simulink model "Design_5new_4weeks"  (R2026a)
settings: Solver=FixedStepAuto  StopTime=200000  FixedStep=300
undefined symbols (not defined in the file): m, n
libraries: mqttlib x7
(part 2 of 2)

== matlab function Design_5new_4weeks/MATLAB Function 3 ==
  data: t input; dt output



function dt = fcn_printer2(t)
%#codegen

SEC_PER_DAY = 24*3600;
rel_sec = 8*3600;    % Same as Printer 1 → 08:00 AM
epsT = 1e-9;

day  = floor(t/SEC_PER_DAY);
tod  = mod(t, SEC_PER_DAY);

next_day = day;

while true
    ndow  = mod(next_day,7);      % day of week
    nweek = floor(next_day/7);    % week index

    % Skip weekends
    if ndow == 5 || ndow == 6
        next_day = next_day + 1;
        continue;
    end

    % Skip first Monday of week 1
    if (nweek == 0) && (ndow == 0)
        next_day = next_day + 1;
        continue;
    end

    % Check today's time
    if next_day == day
        if tod < rel_sec - epsT
            break;   % release today at 08:00
        else
            next_day = next_day + 1;
            continue;
        end
    else
        break;
    end
end

next_release = next_day*SEC_PER_DAY + rel_sec;

% Ensure positive time step
dt = max(next_release - t, 1e-6);

end

== matlab function Design_5new_4weeks/MATLAB Function 4 ==
  data: t input; cap output




function cap = operator_capacity_p2(t)
%#codegen

SEC_PER_DAY = 24*3600;

day = floor(t/SEC_PER_DAY);     % Day index
tod = mod(t, SEC_PER_DAY);      % Time of day (seconds)
dow = mod(day,7);               % Day of week (0=Mon,...,6=Sun)
week = floor(day/7);            % Week index

% --- Weekend: no operator ---
if dow >= 5
    cap = 0;
    return;
end

% --- Special case: First Monday (week 0) ---
if (week == 0) && (dow == 0)
    % Only 12:00–16:00
    if tod >= 12*3600 && tod < 16*3600
        cap = 1;
    else
        cap = 0;
    end
else
    % Normal weekdays: 08:00–16:00
    if tod >= 8*3600 && tod < 16*3600
        cap = 1;
    else
        cap = 0;
    end
end

end

== matlab function Design_5new_4weeks/MATLAB Function 1 ==
  data: t input; dt output



function dt = fcn(t)
%#codegen

SEC_PER_DAY = 24*3600;
rel_sec = 8*3600;      % 08:00
epsT = 1e-9;

day  = floor(t/SEC_PER_DAY);
tod  = mod(t, SEC_PER_DAY);

next_day = day;

while true
    ndow  = mod(next_day,7);
    nweek = floor(next_day/7);

    if ndow == 5 || ndow == 6
        next_day = next_day + 1;
        continue;
    end

    if (nweek == 0) && (ndow == 0)
        next_day = next_day + 1;
        continue;
    end

    if next_day == day
        if tod < rel_sec - epsT
            break;
        else
            next_day = next_day + 1;
            continue;
        end
    else
        break;
    end
end

next_release = next_day*SEC_PER_DAY + rel_sec;
dt = max(next_release - t, 1e-6);

end

== matlab function Design_5new_4weeks/MATLAB Function 2 ==
  data: t input; cap output




function cap = operator_capacity_p1(t)
%#codegen

SEC_PER_DAY = 24*3600;

day = floor(t/SEC_PER_DAY);     % Day index
tod = mod(t, SEC_PER_DAY);      % Time of day (seconds)
dow = mod(day,7);               % Day of week (0=Mon,...,6=Sun)
week = floor(day/7);            % Week index

% --- Weekend: no operator ---
if dow >= 5
    cap = 0;
    return;
end

% --- Special case: First Monday (week 0) ---
if (week == 0) && (dow == 0)
    % Only 12:00–16:00
    if tod >= 12*3600 && tod < 16*3600
        cap = 1;
    else
        cap = 0;
    end
else
    % Normal weekdays: 08:00–16:00
    if tod >= 8*3600 && tod < 16*3600
        cap = 1;
    else
        cap = 0;
    end
end

end

== matlab function Design_5new_4weeks/MATLAB Function manual ==
  data: payload output string
function payload = fcn()
%#codegen

BuildID = 1;
ManualBatchID = 0;
PartID = 5;
Volume = 9.00;
ProcessTime = 30.00;
Energy = 0.000;

payload = string(sprintf( ...
    '[{"BuildID":%.0f},{"ManualBatchID":%.0f},{"PartID":%.0f},{"Volume":%.2f},{"ProcessTime":%.2f},{"Energy":%.3f}]', ...
    BuildID, ManualBatchID, PartID, Volume, ProcessTime, Energy));

end

== matlab function Design_5new_4weeks/Simulink Function Blasting MQTT/MATLAB Function Blasting ==
  data: payload output string; BuildID input; BatchID input; BlastBatchID input; PartID input; Volume input; ProcessTime input; Energy input


function payload = fcn(BuildID,BatchID,BlastBatchID,...
                       PartID,Volume,ProcessTime,Energy)
%#codegen

payload = string(sprintf( ...
    ['[{"BuildID":%.0f},{"BatchID":%.0f},{"BlastBatchID":%.0f},' ...
     '{"PartID":%.0f},{"Volume":%.2f},{"ProcessTime":%.2f},' ...
     '{"Energy":%.3f}]'], ...
    BuildID, BatchID, BlastBatchID, ...
    PartID, Volume, ProcessTime, Energy));

end

== matlab function Design_5new_4weeks/MATLAB Function Surfacing ==
  data: payload output string
function payload = fcn()
%#codegen

BuildID = 1;
BatchID = 9001;
SurfacingBatchID = 9001;
ColoringInputBatchID = 9001;
PartID = 1;
Volume = 5.00;
ProcessTime = 10.00;
Energy = 0.833;

payload = string(sprintf( ...
    '[{"BuildID":%.0f},{"BatchID":%.0f},{"SurfacingBatchID":%.0f},{"ColoringInputBatchID":%.0f},{"PartID":%.0f},{"Volume":%.2f},{"ProcessTime":%.2f},{"Energy":%.3f}]', ...
    BuildID, BatchID, SurfacingBatchID, ColoringInputBatchID, ...
    PartID, Volume, ProcessTime, Energy));

end
